simulink model "GDFLIB_FilterMA_BAM_FLT"  (Simulink 8.3)
settings: Solver=ode45  StartTime=0.0  StopTime=10.0  RelTol=1e-3
undefined symbols (not defined in the file): fltLambda
settings Model: Creator=RE004C  LastModifiedBy=B37097
settings OptimizationCC: ExpressionDepthLimit=2147483647
settings DebuggingCC: FcnCallInpInsideContextMsg=UseLocalSettings  StrictBusMsg=Warning
settings HardwareCC: ProdLargestAtomicInteger=Long  ProdLargestAtomicFloat=Double  ProdIntDivRoundTo=Zero  ProdEndianess=BigEndian  ProdHWDeviceType=Freescale->32-bit PowerPC

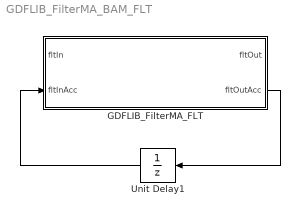
== system GDFLIB_FilterMA_BAM_FLT ==
  GDFLIB_FilterMA_FLT : Subsystem  mask(GDFLIB_FilterMA_FLT){fltLambda=fltLambda}
      mask help: Bit accurate model of exponential moving average filter. All parameters as well as input and output are single precision floating-point values.
      mask init:
      | pos = get_param(gcb, 'Position');width = pos(3) - pos(1); height = pos(4) - pos(2);tX=width/2;tY=height*0.9;
      mask Display:
      | color('black');
      | port_label('input',1,'fltIn');
      | port_label('input',2,'fltInAcc');
      | port_label('output',1,'fltOut');
      | port_label('output',2,'fltOutAcc');
      | color('black');
      | disp('GDFLIB_FilterMA_FLT');
      | color('blue');
      | text(tX,tY, 'BAM', 'horizontalAlignment', 'center');
  Unit Delay1 : UnitDelay  SampleTime=-1
  wires:
  GDFLIB_FilterMA_FLT/2(fltOutAcc) -> Unit Delay1/1
  Unit Delay1/1 -> GDFLIB_FilterMA_FLT/2(fltInAcc)

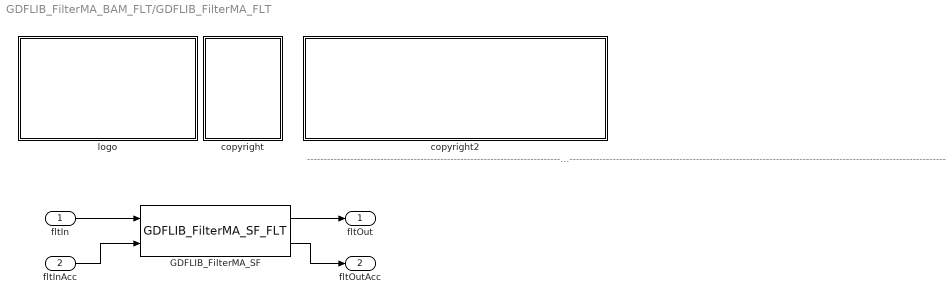
== system GDFLIB_FilterMA_BAM_FLT/GDFLIB_FilterMA_FLT ==
  note: ---------------------------------------------------------------------------------------------------------------------------------------------------------------------------------------------------
  fltIn : Inport
  fltInAcc : Inport  Port=2
  GDFLIB_FilterMA_SF : S-Function  FunctionName=GDFLIB_FilterMA_SF_FLT  Parameters=fltLambda  EnableBusSupport=off
  copyright : Subsystem
      mask Display:
      | text(10,90,'FILE:');text(10,75,'DESRIPTION:')
      | text(10,60,'COPYRIGHT:')
      | text(10,45,'VERSION:')
      | text(10,30,'DATE:')
  copyright2 : Subsystem
      mask Display:
      | text(10,90,'GDFLIB_FilterMA_BAM_FLT.mdl');text(10,75,'Recursive form moving average filter.');text(10,60,'Freescale')
      | text(10,45,'0.1');text(10,30,'16-Jan-2012');
  logo : Subsystem
      mask Display: image(imread('logo.jpg'))
  fltOut : Outport
  fltOutAcc : Outport  Port=2
  wires:
  fltIn/1 -> GDFLIB_FilterMA_SF/1
  GDFLIB_FilterMA_SF/1 -> fltOut/1
  fltInAcc/1 -> GDFLIB_FilterMA_SF/2
  GDFLIB_FilterMA_SF/2 -> fltOutAcc/1

== system GDFLIB_FilterMA_BAM_FLT/GDFLIB_FilterMA_FLT/copyright ==

== system GDFLIB_FilterMA_BAM_FLT/GDFLIB_FilterMA_FLT/copyright2 ==

== system GDFLIB_FilterMA_BAM_FLT/GDFLIB_FilterMA_FLT/logo ==
